simulink model "test_model_2_merging"  (R2020b)
settings: Solver=VariableStepAuto  StartTime=0.0  StopTime=inf  RelTol=1e-3
values from neighbouring files (symbols this model uses):
  AUV = struct    [Parameters_2.m]
  HydroDyn = struct    [Parameters_2.m]
  kc = 57.2958    [Calculations.m]    (also in Parameters_2.m)
  Vfwd = Vfwd(2)    [Parameters_2.m]
  Z_delay = 0.01    [Parameters_2.m]
libraries: slrealtimeutilitieslib x2, slrealtimeiplib x2, sldrtlib x1, simulink x1
settings Model: Creator=117-11  LastModifiedBy=corsair
settings DataIOCC: ReturnWorkspaceOutputs=off
settings DebuggingCC: ArithmeticOperatorsInVariantConditions=warning
settings SFSimCC: CustomCodeUndefinedFunction=UseInterfaceOnly

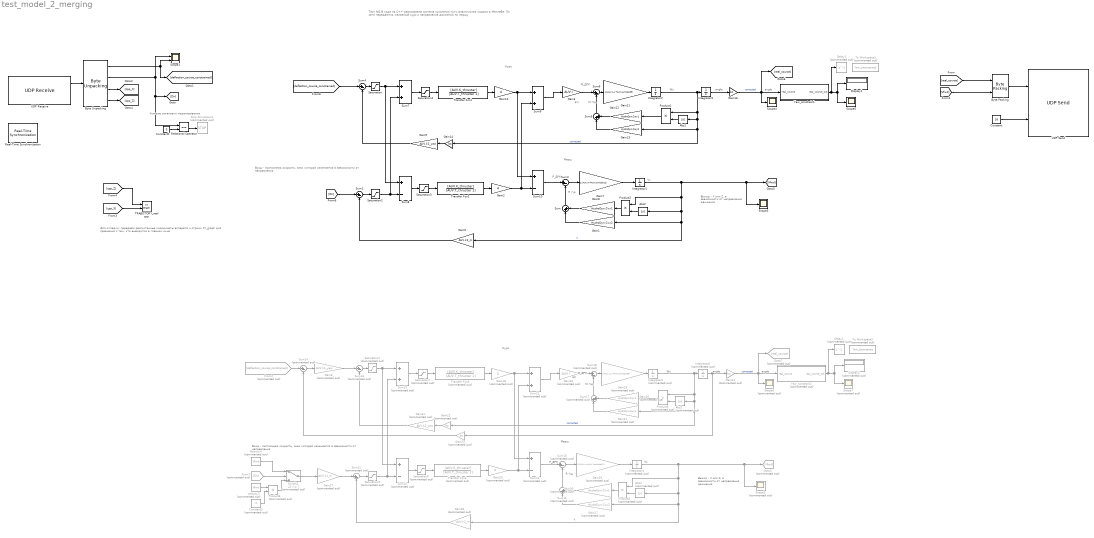
== system test_model_2_merging ==
  note: Тест №2
      |
      | В коде на С++ реализована система счисления пути аналогичная модели в Матлабе.
      | По сети передаются желаемый курс и направление движения по маршу
  note: Условие остановки моделирования
  note: Для отладки: передаём рассчитанные координаты аппарата и строим XY_graph для сравнения с тем, что выводится в главном окне
  note: Курс
  note: 4*l
  note: Марш
  note: angle
  note: R г\д
  note: Wy
  note: P_ДРК
  note: M_ДРК
  note: M г\д
  note: Vx
  note: Выход - X или Z, в зависимости от направления движения
  note: Вход - постоянная скорость, знак которой изменяется в зависимости от направления
  note: angle
  note: Курс
  note: 4*l
  note: Марш
  note: angle
  note: R г\д
  note: Wy
  note: P_ДРК
  note: M_ДРК
  note: M г\д
  note: Vx
  note: Выход - X или Z, в зависимости от направления движения
  note: Вход - постоянная скорость, знак которой изменяется в зависимости от направления
  note: angle
  Abs1 : Abs
  Abs2 : Abs
  Abs3 : Abs  Commented=on
  Abs4 : Abs  Commented=on
  "Byte Packing " : slrealtimeutilitieslib/Byte Packing  MaskPackedDataType=uint8  MaskUnpackedDataTypes={'double', 'double'}  MaskAlignment=1
  "Byte Unpacking " : slrealtimeutilitieslib/Byte Unpacking  MaskUnpackedDataTypes={'double', 'double', 'double', 'double'}  MaskUnpackedDataSizes={[1], [1], [1], [1]}  MaskAlignment=1
      settings: SourceProductBaseCode=XP
  Constant : Constant  Value=16
  Constant1 : Constant  Value=0
  Constant3 : Constant  Commented=on  Value=-1
  Delay1 : Delay  Commented=on  DelayLength=1  InitialCondition=180  SampleTime=Z_delay
  Delay2 : Delay  Commented=on  DelayLength=1  InitialCondition=180  SampleTime=Z_delay
  Display1 : Display
  Display2 : Display  Commented=on
  From2 : From  Commented=on  GotoTag=deflection_course_constrained
  From7 : From  Commented=on  GotoTag=Dir
  Gain1 : Gain  Gain=HydroDyn.Cvx2
  Gain10 : Gain  Gain=4
  Gain11 : Gain  Gain=1/(AUV.Jyy+AUV.lambda55)
  Gain12 : Gain  Gain=HydroDyn.Cwy1
  Gain13 : Gain  Gain=HydroDyn.Cwy2
  Gain14 : Gain  Gain=kc
  Gain16 : Gain  Gain=kc
  Gain17 : Gain  Commented=on  Gain=HydroDyn.Cvx2
  Gain18 : Gain  Commented=on  Gain=4
  Gain19 : Gain  Commented=on  Gain=1/(AUV.Jyy+AUV.lambda55)
  Gain2 : Gain  Gain=4
  Gain20 : Gain  Commented=on  Gain=HydroDyn.Cwy1
  Gain21 : Gain  Commented=on  Gain=HydroDyn.Cwy2
  Gain22 : Gain  Commented=on  Gain=kc
  Gain23 : Gain  Commented=on  Gain=kc
  Gain24 : Gain  Commented=on  Gain=kc
  Gain25 : Gain  Commented=on  Gain=4
  Gain26 : Gain  Commented=on  Gain=AUV.l
  Gain27 : Gain  Commented=on  Gain=AUV.k1_m
  Gain28 : Gain  Commented=on  Gain=AUV.k2_m
  Gain29 : Gain  Commented=on  Gain=1/(AUV.m+AUV.lambda11)
  Gain3 : Gain  Gain=AUV.l
  Gain30 : Gain  Commented=on  Gain=HydroDyn.Cvx1
  Gain31 : Gain  Commented=on  Gain=AUV.k2_yaw
  Gain5 : Gain  Gain=AUV.k2_m
  Gain6 : Gain  Commented=on  Gain=AUV.k1_yaw
  Gain7 : Gain  Gain=1/(AUV.m+AUV.lambda11)
  Gain8 : Gain  Gain=HydroDyn.Cvx1
  Gain9 : Gain  Gain=AUV.k2_yaw
  Goto3 : Goto  Commented=on  GotoTag=Vfwd
  Goto7 : Goto  Commented=on  GotoTag=real_course
  Integrator1 : Integrator  InitialCondition=0.7
  Integrator2 : Integrator
  Integrator3 : Integrator  InitialCondition=3.1416
  Integrator4 : Integrator  Commented=on  InitialCondition=0.7
  Integrator5 : Integrator  Commented=on
  Integrator6 : Integrator  Commented=on  InitialCondition=3.1416
  Product1 : Product
  Product2 : Product
  Product3 : Product  Commented=on
  Product5 : Product  Commented=on
  Product6 : Product  Commented=on
  Real-Time Synchronization : sldrtlib/Real-Time Synchronization  SampleTime=0.001  MaxMissedTicks=10  ShowMissedTicks=off  YieldWhenWaiting=off
  Relational Operator : RelationalOperator  Operator===  OutDataTypeStr=boolean  RndMeth=Simplest
  Saturation : Saturate  UpperLimit=24  LowerLimit=-24
  Saturation1 : Saturate  Commented=on  UpperLimit=24  LowerLimit=-24
  Saturation2 : Saturate  UpperLimit=24  LowerLimit=-24
  Saturation3 : Saturate  UpperLimit=12  LowerLimit=-12
  Saturation4 : Saturate  UpperLimit=12  LowerLimit=-12
  Saturation5 : Saturate  Commented=on  UpperLimit=24  LowerLimit=-24
  Saturation6 : Saturate  Commented=on  UpperLimit=12  LowerLimit=-12
  Saturation7 : Saturate  Commented=on  UpperLimit=12  LowerLimit=-12
  Scope1 : Scope  NumInputPorts=2
  Scope2 : Scope  Commented=on
  Scope3 : Scope
  Scope4 : Scope
  Scope5 : Scope
  Scope6 : Scope  Commented=on
  Scope7 : Scope  Commented=on
  Stop Simulation1 : Stop  Commented=on
  Sum : Sum  Inputs=|++
  Sum{1,3..4,6} (4 alike) : Sum  Inputs=|+-
  Sum10 : Sum  Inputs=+-
  Sum11 : Sum  Commented=on  Inputs=|++
  Sum{12,14..16,18} (5 alike) : Sum  Commented=on  Inputs=|+-
  Sum13 : Sum  Commented=on  Inputs=+-
  Sum17 : Sum  Commented=on  Inputs=|++
  Sum19 : Sum  Commented=on
  Sum20 : Sum  Commented=on  Inputs=+-
  Sum21 : Sum  Commented=on
  Sum5 : Sum  Inputs=|++
  Sum7 : Sum
  Sum8 : Sum  Inputs=+-
  Sum9 : Sum
  Switch2 : Switch  Commented=on  Threshold=1
  TRAJECTORY_real cpp : simulink/Sinks/XY Graph  xmin=-15  xmax=15  ymin=-15  ymax=15  st=Z_delay
  To Workspace1 : ToWorkspace  Commented=on  VariableName=Yaw_tiemseries1  SaveFormat=Timeseries  SampleTime=-1
  To Workspace2 : ToWorkspace  Commented=on  VariableName=Yaw_tiemseries  SaveFormat=Timeseries  SampleTime=-1
  Transfer Fcn1 : TransferFcn  Numerator=[AUV.K_thruster]  Denominator=[AUV.T_thruster 1]
  Transfer Fcn2 : TransferFcn  Numerator=[AUV.K_thruster]  Denominator=[AUV.T_thruster 1]
  Transfer Fcn3 : TransferFcn  Commented=on  Numerator=[AUV.K_thruster]  Denominator=[AUV.T_thruster 1]
  Transfer Fcn4 : TransferFcn  Commented=on  Numerator=[AUV.K_thruster]  Denominator=[AUV.T_thruster 1]
  UDP Receive : slrealtimeiplib/UDP Receive  useHostTargetConn=on  ipAddress=10.10.10.15  localPort=13042  rcvWidth=32  rcvFmAny=on  fmAddress=0.0.0.0  rcvMulticast=off  multicastAddress={}  sampleTime=-1
      settings: SourceProductBaseCode=XP
  UDP Send : slrealtimeiplib/UDP Send  useHostTargetConn=on  ipAddress=10.10.10.15  localPort=13043  toAddress=127.0.0.1  toPort=13044  sampleTime=0.001
      settings: SourceProductBaseCode=XP
  Velocity3 : Constant  Commented=on  Value=Vfwd
  Velocity4 : Constant  Commented=on  Value=Vfwd
  Yaw_constrain1 : MATLAB Function  TreatAsAtomicUnit=on
  Yaw_constrain2 : MATLAB Function  Commented=on  TreatAsAtomicUnit=on
  wires:
  "Byte Unpacking "/1 -> [deflection_course_constrained], Scope1/2
  UDP Receive/1 -> "Byte Unpacking "/1
  [real_course] -> "Byte Packing "/1
  Constant/1 -> UDP Send/2
  "Byte Packing "/1 -> UDP Send/1
  "Byte Unpacking "/2 -> Relational Operator/1, [Dir], Scope1/1
  [Vfwd] -> "Byte Packing "/2
  Relational Operator/1 -> Stop Simulation1/1
  Constant1/1 -> Relational Operator/2
  "Byte Unpacking "/3 -> [cpp_X]
  "Byte Unpacking "/4 -> [cpp_Z]
  [cpp_X] -> TRAJECTORY_real cpp/2
  [cpp_Z] -> TRAJECTORY_real cpp/1
  Sum1/1 -> Saturation2/1
  Sum7/1 -> Saturation4/1
  Sum8/1 -> Saturation3/1
  Gain14/1 -> Gain9/1
  [deflection_course_constrained] -> Sum4/1
  Product2/1 -> Gain8/1
  Saturation3/1 -> Transfer Fcn2/1
  Sum3/1 -> Gain7/1
  Gain8/1 -> Sum/2
  Abs1/1 -> Product1/2
  Gain7/1 -> Integrator1/1
  Gain9/1 -> Sum4/2
  Integrator3/1 -> Gain16/1
  Gain3/1 -> Sum6/1
  Gain1/1 -> Sum/1
  Sum5/1 -> Sum6/2
  Sum6/1 -> Gain11/1
  Gain13/1 -> Sum5/1
  Gain12/1 -> Sum5/2
  Gain11/1 -> Integrator2/1
  Sum/1 -> Sum3/2
  Integrator2/1 -> Integrator3/1, Abs1/1, Gain14/1, Gain13/1, Product1/1  "corrected"
  Sum4/1 -> Saturation/1
  Transfer Fcn1/1 -> Gain10/1
  Product1/1 -> Gain12/1
  Sum10/1 -> Sum3/1
  Saturation4/1 -> Transfer Fcn1/1
  Abs2/1 -> Product2/2
  Gain10/1 -> Sum9/1, Sum10/1
  Gain16/1 -> Scope4/1, [real_course], Yaw_constrain1/1(real_course)  "corrected"
  Gain5/1 -> Sum1/2
  Transfer Fcn2/1 -> Gain2/1
  Gain2/1 -> Sum9/2, Sum10/2
  Saturation2/1 -> Sum7/2, Sum8/2
  Saturation/1 -> Sum8/1, Sum7/1
  [Dir] -> Sum1/1
  Sum9/1 -> Gain3/1
  Integrator1/1 -> [Vfwd], Scope3/1, Gain5/1, Gain1/1, Abs2/1, Product2/1  "V"
  Yaw_constrain1/1(real_course_out) -> Delay2/1, Scope5/1, Display1/1
  Yaw_constrain2/1(real_course_out) -> Display2/1, Scope7/1, Delay1/1
  Integrator4/1 -> Product5/1, Abs4/1, Gain17/1, Gain28/1, Scope2/1, Goto3/1  "V"
  Product6/1 -> Switch2/3
  Velocity3/1 -> Product6/1
  Velocity4/1 -> Switch2/1
  Constant3/1 -> Product6/2
  From7/1 -> Switch2/2
  Sum21/1 -> Gain26/1
  Gain27/1 -> Sum12/1
  Saturation1/1 -> Sum19/1, Sum20/1
  Saturation5/1 -> Sum20/2, Sum19/2
  Gain25/1 -> Sum13/2, Sum21/2
  Transfer Fcn4/1 -> Gain25/1
  Gain28/1 -> Sum12/2
  Gain24/1 -> Yaw_constrain2/1(real_course), Goto7/1, Scope6/1  "corrected"
  Sum14/1 -> Gain6/1
  Gain18/1 -> Sum13/1, Sum21/1
  Abs4/1 -> Product5/2
  Saturation7/1 -> Transfer Fcn3/1
  Sum13/1 -> Sum15/1
  Product3/1 -> Gain20/1
  Transfer Fcn3/1 -> Gain18/1
  From2/1 -> Sum14/1
  Sum16/1 -> Saturation1/1
  Integrator5/1 -> Product3/1, Gain21/1, Gain22/1, Abs3/1, Integrator6/1  "corrected"
  Sum11/1 -> Sum15/2
  Gain19/1 -> Integrator5/1
  Gain23/1 -> Sum14/2
  Gain20/1 -> Sum17/2
  Gain21/1 -> Sum17/1
  Sum18/1 -> Gain19/1
  Sum17/1 -> Sum18/2
  Gain17/1 -> Sum11/1
  Gain26/1 -> Sum18/1
  Integrator6/1 -> Gain23/1, Gain24/1
  Gain31/1 -> Sum16/2
  Gain29/1 -> Integrator4/1
  Abs3/1 -> Product3/2
  Gain30/1 -> Sum11/2
  Sum15/1 -> Gain29/1
  Saturation6/1 -> Transfer Fcn4/1
  Switch2/1 -> Gain27/1
  Product5/1 -> Gain30/1
  Gain6/1 -> Sum16/1
  Gain22/1 -> Gain31/1
  Sum20/1 -> Saturation6/1
  Sum19/1 -> Saturation7/1
  Sum12/1 -> Saturation5/1

== matlab function test_model_2_merging/Yaw_constrain1 ==
  data: real_course input; real_course_out output
function real_course_out   = fcn(real_course)

    % Приводим к стандарту
    if real_course < 0
        real_course_out = 360 - abs(real_course);
    elseif real_course >= 360
        real_course_out = real_course - 360;
    else    
        real_course_out = real_course;
    end

end

== matlab function test_model_2_merging/Yaw_constrain2 ==
  data: real_course input; real_course_out output
function real_course_out   = fcn(real_course)

    % Приводим к стандарту
    if real_course < 0
        real_course_out = 360 - abs(real_course);
    elseif real_course >= 360
        real_course_out = real_course - 360;
    else    
        real_course_out = real_course;
    end

end
